simulink model "Pacemaker_Assignment_2_Final"  (R2018b)
settings: Solver=FixedStepAuto  StartTime=0.0  StopTime=inf  FixedStep=1e-3  RelTol=1e-3  EnableMultiTasking=on
undefined symbols (not defined in the file): D0, D1, D10, D11, D12, D13, D2, D3, D4, D5, D6, D7, D8, D9, PTA0, PTA1, PTA2, PTB23, PTB9, PTC16, PTC17, PTC2, PTC3, PTC4, PTD0, PTD1, PTD2, PTD3
libraries: frdmk64flib x20, dspstat3 x1
(part 1 of 2)
settings Model: EnablePacing=on  ExtModeTrigDuration=5  Creator=joelh  LastModifiedBy=joelh
settings OptimizationCC: EnhancedBackFolding=on  PassReuseOutputArgsAs=Individual arguments  MaxStackSize=64  OptimizeBlockOrder=speed  DifferentSizesBufferReuse=on  OptimizationCustomize=off
settings DebuggingCC: ParameterTunabilityLossMsg=error
settings HardwareCC: ProdBitPerPointer=32  ProdBitPerSizeT=32  ProdBitPerPtrDiffT=32  ProdLargestAtomicInteger=Long  ProdLargestAtomicFloat=Double  ProdWordSize=32  ProdHWDeviceType=ARM Compatible->ARM Cortex
settings SFSimCC: MATLABDynamicMemAlloc=off
settings RTWCC: SystemTargetFile=ert.tlc  HardwareBoard=NXP FRDM-K64F  TLCOptions="-aInlineSetEventsForThisBaseRateFcn=TLC_FALSE -aSuppressMultiTaskScheduler=TLC_FALSE  -aRateBasedStepFcn=0"  TemplateMakefile=ert_default_tmf  GenerateReport=on  Toolchain=GNU Tools for ARM Embedded Processors  IncludeHyperlinkInReport=on  LaunchReport=on  GenerateTraceInfo=on  GenerateTraceReport=on  GenerateTraceReportSl=on  GenerateTraceReportSf=on  GenerateTraceReportEml=on
settings CodeAppCC: ForceParamTrailComments=on  IgnoreCustomStorageClasses=off  OperatorAnnotations=on  SimulinkDataObjDesc=on  SFDataObjDesc=on  InsertBlockDesc=on

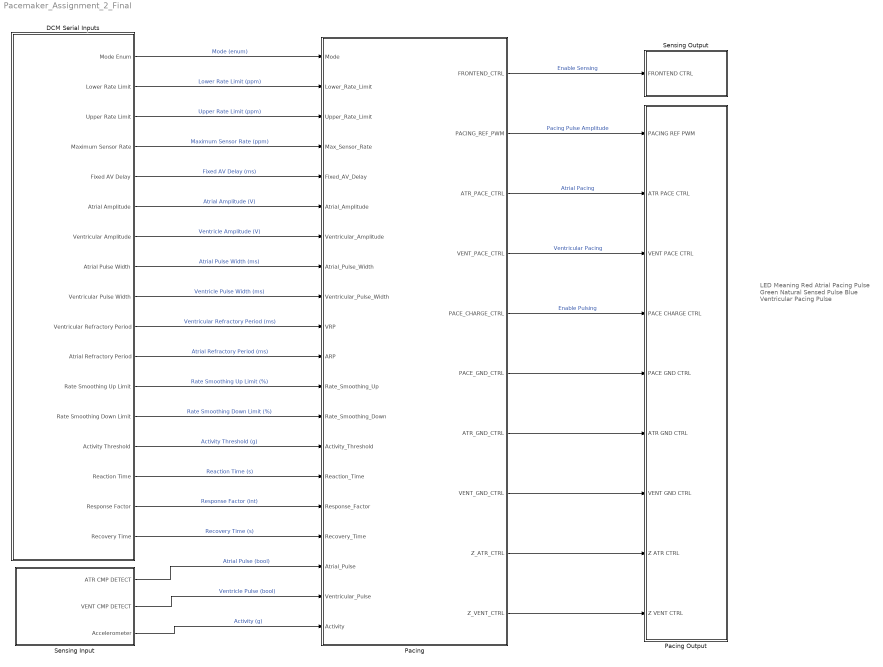
== system Pacemaker_Assignment_2_Final ==
  note: LED
      | Meaning
      |
      | Red
      | Atrial Pacing Pulse
      |
      | Green
      | Natural Sensed Pulse
      |
      | Blue
      | Ventricular Pacing Pulse
  DCM Serial Inputs : Subsystem
  Pacing : Stateflow chart  TreatAsAtomicUnit=on
  Pacing Output : Subsystem
  Sensing Input : Subsystem
  Sensing Output : Subsystem
  wires:
  DCM Serial Inputs/1(Mode Enum) -> Pacing/1(Mode)  "Mode (enum)"
  DCM Serial Inputs/2(Lower Rate Limit) -> Pacing/2(Lower_Rate_Limit)  "Lower Rate Limit (ppm)"
  DCM Serial Inputs/3(Upper Rate Limit) -> Pacing/3(Upper_Rate_Limit)  "Upper Rate Limit (ppm)"
  DCM Serial Inputs/4(Maximum Sensor Rate) -> Pacing/4(Max_Sensor_Rate)  "Maximum Sensor Rate (ppm)"
  DCM Serial Inputs/5(Fixed AV Delay) -> Pacing/5(Fixed_AV_Delay)  "Fixed AV Delay (ms)"
  DCM Serial Inputs/6(Atrial Amplitude) -> Pacing/6(Atrial_Amplitude)  "Atrial Amplitude (V)"
  DCM Serial Inputs/7(Ventricular Amplitude) -> Pacing/7(Ventricular_Amplitude)  "Ventricle Amplitude (V)"
  DCM Serial Inputs/8(Atrial Pulse Width) -> Pacing/8(Atrial_Pulse_Width)  "Atrial Pulse Width (ms)"
  DCM Serial Inputs/9(Ventricular Pulse Width) -> Pacing/9(Ventricular_Pulse_Width)  "Ventricle Pulse Width (ms)"
  DCM Serial Inputs/10(Ventricular Refractory Period) -> Pacing/10(VRP)  "Ventricular Refractory Period (ms)"
  DCM Serial Inputs/11(Atrial Refractory Period) -> Pacing/11(ARP)  "Atrial Refractory Period (ms)"
  DCM Serial Inputs/12(Rate Smoothing Up Limit) -> Pacing/12(Rate_Smoothing_Up)  "Rate Smoothing Up Limit (%)"
  DCM Serial Inputs/13(Rate Smoothing Down Limit) -> Pacing/13(Rate_Smoothing_Down)  "Rate Smoothing Down Limit (%)"
  DCM Serial Inputs/14(Activity Threshold) -> Pacing/14(Activity_Threshold)  "Activity Threshold (g)"
  DCM Serial Inputs/15(Reaction Time) -> Pacing/15(Reaction_Time)  "Reaction Time (s)"
  DCM Serial Inputs/16(Response Factor) -> Pacing/16(Response_Factor)  "Response Factor (int)"
  DCM Serial Inputs/17(Recovery Time) -> Pacing/17(Recovery_Time)  "Recovery Time (s)"
  Sensing Input/1(ATR CMP DETECT) -> Pacing/18(Atrial_Pulse)  "Atrial Pulse (bool)"
  Sensing Input/2(VENT CMP DETECT) -> Pacing/19(Ventricular_Pulse)  "Ventricle Pulse (bool)"
  Sensing Input/3(Accelerometer) -> Pacing/20(Activity)  "Activity (g)"
  Pacing/1(FRONTEND_CTRL) -> Sensing Output/1(FRONTEND CTRL)  "Enable Sensing"
  Pacing/2(PACING_REF_PWM) -> Pacing Output/1(PACING REF PWM)  "Pacing Pulse Amplitude"
  Pacing/3(ATR_PACE_CTRL) -> Pacing Output/2(ATR PACE CTRL)  "Atrial Pacing"
  Pacing/4(VENT_PACE_CTRL) -> Pacing Output/3(VENT PACE CTRL)  "Ventricular Pacing"
  Pacing/5(PACE_CHARGE_CTRL) -> Pacing Output/4(PACE CHARGE CTRL)  "Enable Pulsing"
  Pacing/6(PACE_GND_CTRL) -> Pacing Output/5(PACE GND CTRL)
  Pacing/7(ATR_GND_CTRL) -> Pacing Output/6(ATR GND CTRL)
  Pacing/8(VENT_GND_CTRL) -> Pacing Output/7(VENT GND CTRL)
  Pacing/9(Z_ATR_CTRL) -> Pacing Output/8(Z ATR CTRL)
  Pacing/10(Z_VENT_CTRL) -> Pacing Output/9(Z VENT CTRL)

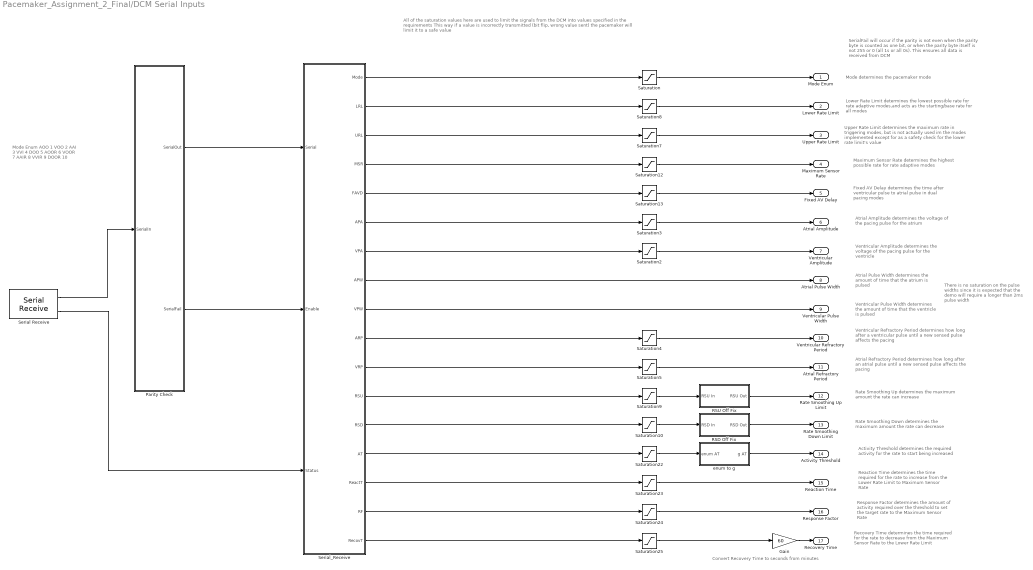
== system Pacemaker_Assignment_2_Final/DCM Serial Inputs ==
  note: Convert Recovery Time to seconds from minutes
  note: Recovery Time determines the time required for the rate to decrease from
      | the Maximum Sensor Rate to the Lower Rate Limit
  note: Response Factor determines the amount of activity required over the threshold to set the target rate to the Maximum Sensor Rate
  note: Reaction Time determines the time required for the rate to increase from the Lower Rate Limit to Maximum Sensor Rate
  note: Activity Threshold determines the required activity for the rate to start being increased
  note: Rate Smoothing Up determines the maximum amount the rate can increase
  note: Ventricular Refractory Period determines how long after a ventricular pulse until a new sensed pulse affects the pacing
  note: There is no saturation on the pulse widths since it is expected that
      | the demo will require a longer than 2ms pulse width
  note: Atrial Pulse Width determines the amount of time that the atrium is pulsed
  note: Atrial Amplitude determines the voltage of the pacing pulse for the atrium
  note: Fixed AV Delay determines the time after ventricular pulse to atrial pulse in
      | dual pacing modes
  note: Maximum Sensor Rate determines the highest possible rate for rate adaptive modes
  note: Upper Rate Limit determines the maximum rate in triggering modes, but is not actually used im the modes implemented except for as a safety check for the lower rate limit's value
  note: Lower Rate Limit determines the lowest possible rate for rate adaptive modes,and acts as the starting/base rate for all modes
  note: SerialFail will occur if the parity is not even when the parity byte is counted as one bit, or when the parity byte itself is not 255 or 0 (all 1s or all 0s). This ensures all data is received from DCM
  note: Mode determines the pacemaker mode
  note: All of the saturation values here are used to limit the signals from the DCM into values specified in the requirements
      | This way if a value is incorrectly transmitted (bit flip, wrong value sent) the pacemaker will limit it to a safe value
  note: Mode
      | Enum
      |
      | AOO
      | 1
      |
      | VOO
      | 2
      |
      | AAI
      | 3
      |
      | VVI
      | 4
      |
      | DOO
      | 5
      |
      | AOOR
      | 6
      |
      | VOOR
      | 7
      |
      | AAIR
      | 8
      |
      | VVIR
      | 9
      |
      | DOOR
      | 10
  note: Ventricular Amplitude determines the voltage of the pacing pulse for the ventricle
  note: Ventricular Pulse Width determines the amount of time that the ventricle is pulsed
  note: Atrial Refractory Period determines how long after an atrial pulse until a new sensed pulse affects the pacing
  note: Rate Smoothing Down determines the maximum amount the rate can decrease
  Gain : Gain  Gain=60
  Parity Check : MATLAB Function  TreatAsAtomicUnit=on
  RSD Off Fix : Subsystem
  RSU Off Fix : Subsystem
  Saturation : Saturate  UpperLimit=10  LowerLimit=0
  Saturation10 : Saturate  UpperLimit=25  LowerLimit=0
  Saturation12 : Saturate  UpperLimit=175  LowerLimit=50
  Saturation13 : Saturate  UpperLimit=300  LowerLimit=70
  Saturation2 : Saturate  UpperLimit=5  LowerLimit=0
  Saturation22 : Saturate  UpperLimit=7  LowerLimit=1
  Saturation23 : Saturate  UpperLimit=50  LowerLimit=10
  Saturation24 : Saturate  UpperLimit=16  LowerLimit=1
  Saturation25 : Saturate  UpperLimit=16  LowerLimit=2
  Saturation3 : Saturate  UpperLimit=5  LowerLimit=0
  Saturation4 : Saturate  UpperLimit=500  LowerLimit=150
  Saturation5 : Saturate  UpperLimit=500  LowerLimit=150
  Saturation7 : Saturate  UpperLimit=175  LowerLimit=50
  Saturation8 : Saturate  UpperLimit=175  LowerLimit=30
  Saturation9 : Saturate  UpperLimit=25  LowerLimit=0
  Serial Receive : frdmk64flib/Serial Receive  SCIModule=0  Baudrate=uint32(9600)  Parity=None  StopBits=1  HardwareFlowControl=None  ByteOrder=LittleEndian  DataType=uint8  DataLength=18  BlockingMode=off  OutputStatus=on  SampleTime=-1
      settings: SourceProductName=Simulink Coder Support Package for NXP FRDM-K64F Board
  Serial_Receive : Stateflow chart  TreatAsAtomicUnit=on
  enum to g : Subsystem
  Mode Enum : Outport
  Lower Rate Limit : Outport  Port=2
  Upper Rate Limit : Outport  Port=3
  Maximum Sensor Rate : Outport  Port=4
  Fixed AV Delay : Outport  Port=5
  Atrial Amplitude : Outport  Port=6
  Ventricular Amplitude : Outport  Port=7
  Atrial Pulse Width : Outport  Port=8
  Ventricular Pulse Width : Outport  Port=9
  Ventricular Refractory Period : Outport  Port=10
  Atrial Refractory Period : Outport  Port=11
  Rate Smoothing Up Limit : Outport  Port=12
  Rate Smoothing Down Limit : Outport  Port=13
  Activity Threshold : Outport  Port=14
  Reaction Time : Outport  Port=15
  Response Factor : Outport  Port=16
  Recovery Time : Outport  Port=17
  wires:
  Serial_Receive/6(APA) -> Saturation3/1
  Serial_Receive/2(LRL) -> Saturation8/1
  Serial_Receive/7(VPA) -> Saturation2/1
  Serial_Receive/3(URL) -> Saturation7/1
  Serial_Receive/10(ARP) -> Saturation4/1
  Serial_Receive/11(VRP) -> Saturation5/1
  Serial_Receive/12(RSU) -> Saturation9/1
  Serial_Receive/13(RSD) -> Saturation10/1
  Saturation2/1 -> Ventricular Amplitude/1
  Saturation3/1 -> Atrial Amplitude/1
  Saturation4/1 -> Ventricular Refractory Period/1
  Saturation5/1 -> Atrial Refractory Period/1
  Saturation7/1 -> Upper Rate Limit/1
  Saturation8/1 -> Lower Rate Limit/1
  Saturation9/1 -> RSU Off Fix/1(RSU In)
  Saturation10/1 -> RSD Off Fix/1(RSD In)
  Serial_Receive/5(FAVD) -> Saturation13/1
  Serial_Receive/4(MSR) -> Saturation12/1
  Serial_Receive/14(AT) -> Saturation22/1
  Serial_Receive/15(ReactT) -> Saturation23/1
  Serial_Receive/16(RF) -> Saturation24/1
  Serial_Receive/17(RecovT) -> Saturation25/1
  Saturation22/1 -> enum to g/1(enum AT)
  Serial_Receive/1(Mode) -> Saturation/1
  Gain/1 -> Recovery Time/1
  Saturation12/1 -> Maximum Sensor Rate/1
  Saturation13/1 -> Fixed AV Delay/1
  Serial_Receive/8(APW) -> Atrial Pulse Width/1
  Serial_Receive/9(VPW) -> Ventricular Pulse Width/1
  Saturation23/1 -> Reaction Time/1
  Saturation24/1 -> Response Factor/1
  Saturation25/1 -> Gain/1
  enum to g/1(g AT) -> Activity Threshold/1
  Saturation/1 -> Mode Enum/1
  Parity Check/1(SerialOut) -> Serial_Receive/1(Serial)
  Serial Receive/1 -> Parity Check/1(SerialIn)
  Serial Receive/2 -> Serial_Receive/3(Status)
  Parity Check/2(SerialFail) -> Serial_Receive/2(Enable)
  RSU Off Fix/1(RSU Out) -> Rate Smoothing Up Limit/1
  RSD Off Fix/1(RSD Out) -> Rate Smoothing Down Limit/1

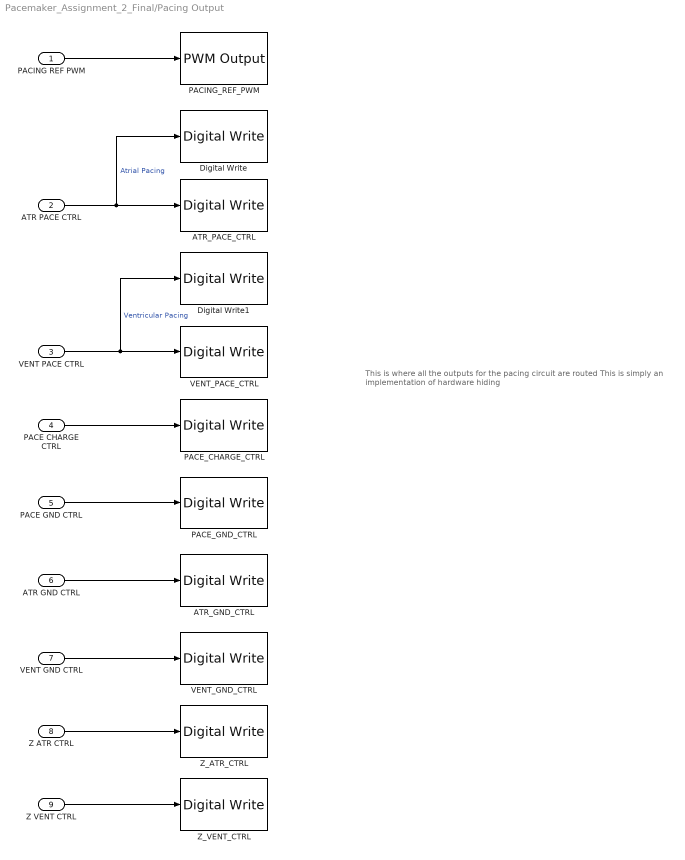
== system Pacemaker_Assignment_2_Final/Pacing Output ==
  note: This is where all the outputs for the pacing circuit are routed
      | This is simply an implementation of hardware hiding
  PACING REF PWM : Inport
  ATR PACE CTRL : Inport  Port=2
  VENT PACE CTRL : Inport  Port=3
  PACE CHARGE CTRL : Inport  Port=4
  PACE GND CTRL : Inport  Port=5
  ATR GND CTRL : Inport  Port=6
  VENT GND CTRL : Inport  Port=7
  Z ATR CTRL : Inport  Port=8
  Z VENT CTRL : Inport  Port=9
  ATR_GND_CTRL : frdmk64flib/Digital Write  Whichpin=PTD2 (D11)
      settings: SourceProductName=Simulink Coder Support Package for NXP FRDM-K64F Board
  ATR_PACE_CTRL : frdmk64flib/Digital Write  Whichpin=PTA0 (D8)
      settings: SourceProductName=Simulink Coder Support Package for NXP FRDM-K64F Board
  Digital Write : frdmk64flib/Digital Write  Whichpin=RED_LED
      settings: SourceProductName=Simulink Coder Support Package for NXP FRDM-K64F Board
  Digital Write1 : frdmk64flib/Digital Write  Whichpin=BLUE_LED
      settings: SourceProductName=Simulink Coder Support Package for NXP FRDM-K64F Board
  PACE_CHARGE_CTRL : frdmk64flib/Digital Write  Whichpin=PTB9 (D2)
      settings: SourceProductName=Simulink Coder Support Package for NXP FRDM-K64F Board
  PACE_GND_CTRL : frdmk64flib/Digital Write  Whichpin=PTD0 (D10)
      settings: SourceProductName=Simulink Coder Support Package for NXP FRDM-K64F Board
  PACING_REF_PWM : frdmk64flib/PWM Output  Whichpin=PTA2 (D5)  InitialFrequency=2000  InitialDutyCycle=0
      settings: SourceProductName=Simulink Coder Support Package for NXP FRDM-K64F Board
  VENT_GND_CTRL : frdmk64flib/Digital Write  Whichpin=PTD3 (D12)
      settings: SourceProductName=Simulink Coder Support Package for NXP FRDM-K64F Board
  VENT_PACE_CTRL : frdmk64flib/Digital Write  Whichpin=PTC4 (D9)
      settings: SourceProductName=Simulink Coder Support Package for NXP FRDM-K64F Board
  Z_ATR_CTRL : frdmk64flib/Digital Write  Whichpin=PTB23 (D4)
      settings: SourceProductName=Simulink Coder Support Package for NXP FRDM-K64F Board
  Z_VENT_CTRL : frdmk64flib/Digital Write  Whichpin=PTC3 (D7)
      settings: SourceProductName=Simulink Coder Support Package for NXP FRDM-K64F Board
  wires:
  ATR GND CTRL/1 -> ATR_GND_CTRL/1
  VENT GND CTRL/1 -> VENT_GND_CTRL/1
  ATR PACE CTRL/1 -> Digital Write/1, ATR_PACE_CTRL/1  "Atrial Pacing"
  PACE GND CTRL/1 -> PACE_GND_CTRL/1
  PACING REF PWM/1 -> PACING_REF_PWM/1
  PACE CHARGE CTRL/1 -> PACE_CHARGE_CTRL/1
  Z ATR CTRL/1 -> Z_ATR_CTRL/1
  Z VENT CTRL/1 -> Z_VENT_CTRL/1
  VENT PACE CTRL/1 -> Digital Write1/1, VENT_PACE_CTRL/1  "Ventricular Pacing"

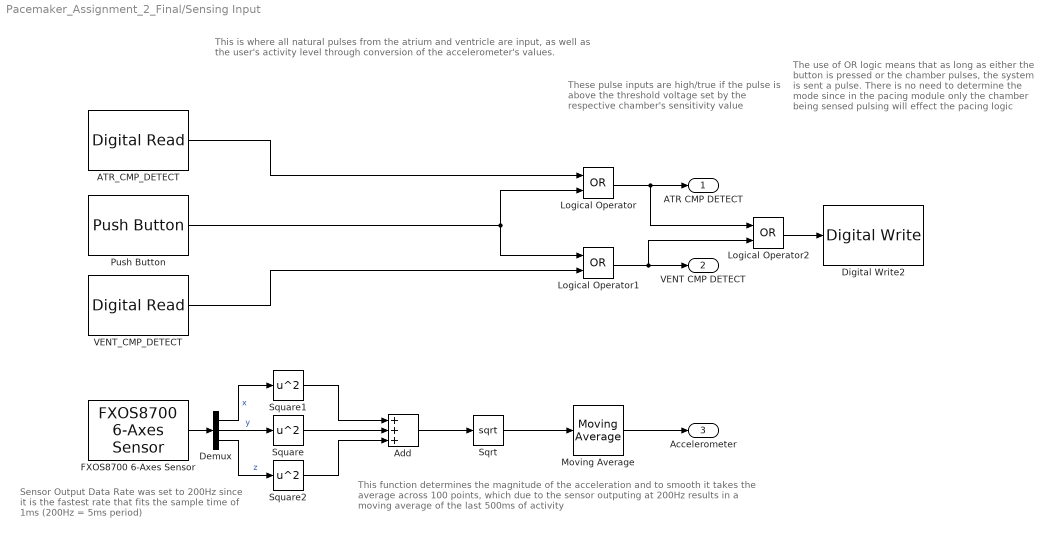
== system Pacemaker_Assignment_2_Final/Sensing Input ==
  note: Sensor Output Data Rate was set to 200Hz since it is the fastest rate that fits the sample time of 1ms (200Hz = 5ms period)
  note: This function determines the magnitude of the acceleration and to smooth it takes the average across 100 points, which due to the sensor outputing at 200Hz results in a moving average of the last 500ms of activity
  note: This is where all natural pulses from the atrium and ventricle are input, as well
      | as the user's activity level through conversion of the accelerometer's values.
  note: The use of OR logic means that as long as either the button is pressed or the chamber pulses, the system is sent a pulse. There is no need to determine the mode since in the pacing module only the chamber being sensed pulsing will effect the pacing logic
  note: These pulse inputs are high/true if the pulse is above the threshold voltage set by the respective chamber's sensitivity value
  ATR_CMP_DETECT : frdmk64flib/Digital Read  Whichpin=PTC16 (D0)  SampleTime=-1
      settings: SourceProductName=Simulink Coder Support Package for NXP FRDM-K64F Board
  Add : Sum  Inputs=3
  Demux : Demux  Outputs=3
  Digital Write2 : frdmk64flib/Digital Write  Whichpin=GREEN_LED
      settings: SourceProductName=Simulink Coder Support Package for NXP FRDM-K64F Board
  FXOS8700 6-Axes Sensor : frdmk64flib/FXOS8700 6-Axes Sensor  Activesensor=Accelerometer only  ODR=200Hz  HybridODR=400Hz  Accelfullrange=-4g to +4g  SampleTime=-1
      settings: SourceProductName=Simulink Coder Support Package for NXP FRDM-K64F Board
  Logical Operator : Logic  Operator=OR  AllPortsSameDT=off  OutDataTypeStr=boolean
  Logical Operator1 : Logic  Operator=OR  AllPortsSameDT=off  OutDataTypeStr=boolean
  Logical Operator2 : Logic  Operator=OR  AllPortsSameDT=off  OutDataTypeStr=boolean
  Moving Average : dspstat3/Moving Average  Method=Sliding window  ForgettingFactorPort=off  SpecifyWindowLength=on  WindowLength=100  ForgettingFactor=0.9  SimulateUsing=Code generation
  "Push Button " : frdmk64flib/Push Button  Whichswitch=SW3  SampleTime1=-1
      settings: SourceProductName=Simulink Coder Support Package for NXP FRDM-K64F Board
  Sqrt : Sqrt  SaturateOnIntegerOverflow=on
  Square : Math  Operator=square  SaturateOnIntegerOverflow=on
  Square1 : Math  Operator=square  SaturateOnIntegerOverflow=on
  Square2 : Math  Operator=square  SaturateOnIntegerOverflow=on
  VENT_CMP_DETECT : frdmk64flib/Digital Read  Whichpin=PTC17 (D1)  SampleTime=-1
      settings: SourceProductName=Simulink Coder Support Package for NXP FRDM-K64F Board
  ATR CMP DETECT : Outport
  VENT CMP DETECT : Outport  Port=2
  Accelerometer : Outport  Port=3
  wires:
  Logical Operator1/1 -> Logical Operator2/2, VENT CMP DETECT/1
  Logical Operator/1 -> Logical Operator2/1, ATR CMP DETECT/1
  ATR_CMP_DETECT/1 -> Logical Operator/1
  "Push Button "/1 -> Logical Operator1/1, Logical Operator/2
  VENT_CMP_DETECT/1 -> Logical Operator1/2
  Moving Average/1 -> Accelerometer/1
  Demux/2 -> Square/1  "y"
  Demux/1 -> Square1/1  "x"
  Add/1 -> Sqrt/1
  FXOS8700 6-Axes Sensor/1 -> Demux/1
  Square/1 -> Add/2
  Square1/1 -> Add/1
  Square2/1 -> Add/3
  Demux/3 -> Square2/1  "z"
  Sqrt/1 -> Moving Average/1
  Logical Operator2/1 -> Digital Write2/1

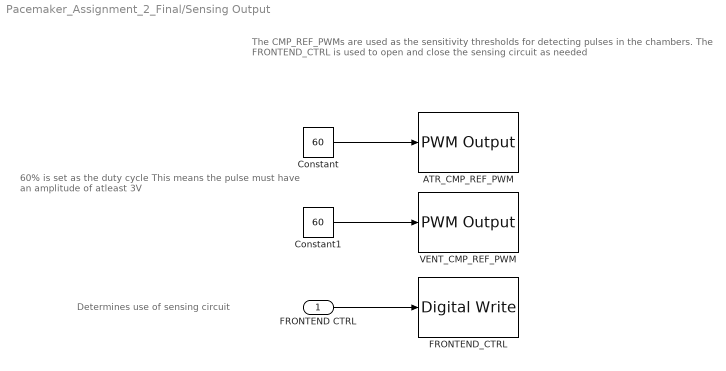
== system Pacemaker_Assignment_2_Final/Sensing Output ==
  note: 60% is set as the duty cycle
      | This means the pulse must have an amplitude of atleast 3V
  note: The CMP_REF_PWMs are used as the sensitivity thresholds for detecting pulses in the chambers.
      | The FRONTEND_CTRL is used to open and close the sensing circuit as needed
  note: Determines use of sensing circuit
  FRONTEND CTRL : Inport
  ATR_CMP_REF_PWM : frdmk64flib/PWM Output  Whichpin=PTC2 (D6)  InitialFrequency=2000  InitialDutyCycle=0
      settings: SourceProductName=Simulink Coder Support Package for NXP FRDM-K64F Board
  Constant : Constant  Value=60
  Constant1 : Constant  Value=60
  FRONTEND_CTRL : frdmk64flib/Digital Write  Whichpin=PTD1 (D13)
      settings: SourceProductName=Simulink Coder Support Package for NXP FRDM-K64F Board
  VENT_CMP_REF_PWM : frdmk64flib/PWM Output  Whichpin=PTA1 (D3)  InitialFrequency=2000  InitialDutyCycle=0
      settings: SourceProductName=Simulink Coder Support Package for NXP FRDM-K64F Board
  wires:
  FRONTEND CTRL/1 -> FRONTEND_CTRL/1
  Constant/1 -> ATR_CMP_REF_PWM/1
  Constant1/1 -> VENT_CMP_REF_PWM/1

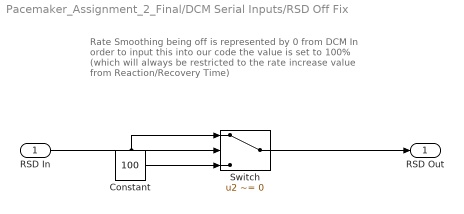
== system Pacemaker_Assignment_2_Final/DCM Serial Inputs/RSD Off Fix ==
  note: Rate Smoothing being off is represented by 0 from DCM
      | In order to input this into our code the value is set to 100% (which will always be restricted to the
      | rate increase value from Reaction/Recovery Time)
  RSD In : Inport
  Constant : Constant  Value=100
  Switch : Switch  Criteria=u2 ~= 0
  RSD Out : Outport
  wires:
  Constant/1 -> Switch/3
  RSD In/1 -> Switch/1, Switch/2
  Switch/1 -> RSD Out/1

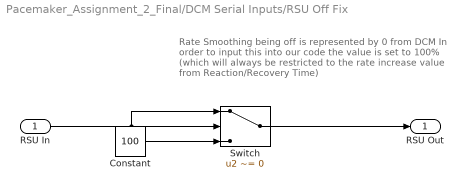
== system Pacemaker_Assignment_2_Final/DCM Serial Inputs/RSU Off Fix ==
  note: Rate Smoothing being off is represented by 0 from DCM
      | In order to input this into our code the value is set to 100% (which will always be restricted to the
      | rate increase value from Reaction/Recovery Time)
  RSU In : Inport
  Constant : Constant  Value=100
  Switch : Switch  Criteria=u2 ~= 0
  RSU Out : Outport
  wires:
  RSU In/1 -> Switch/1, Switch/2
  Switch/1 -> RSU Out/1
  Constant/1 -> Switch/3

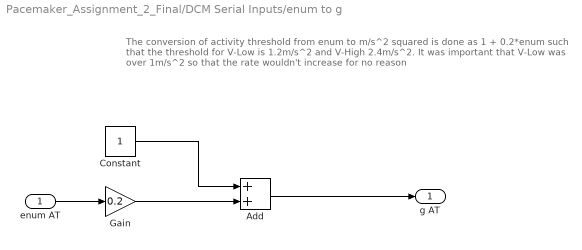
== system Pacemaker_Assignment_2_Final/DCM Serial Inputs/enum to g ==
  note: The conversion of activity threshold from enum to m/s^2 squared is done as
      | 1 + 0.2*enum such that the threshold for V-Low is 1.2m/s^2 and V-High 2.4m/s^2.
      | It was important that V-Low was over 1m/s^2 so that the rate wouldn't increase for no reason
  enum AT : Inport
  Add : Sum
  Constant : Constant
  Gain : Gain  Gain=0.2
  g AT : Outport
  wires:
  enum AT/1 -> Gain/1
  Gain/1 -> Add/2
  Add/1 -> g AT/1
  Constant/1 -> Add/1

== matlab function Pacemaker_Assignment_2_Final/DCM Serial Inputs/Parity Check ==
  data: SerialOut output uint8; SerialFail output boolean; SerialIn input
function [SerialOut, SerialFail]= Unpack(SerialIn)
%This is the serial checking and unpacking of the parameters from DCM
%Byte 1: Parity (SerialFail) Using Even parity
if (SerialIn(1) == 255) %Odd number of 1s in bytes 2-18
    numOnes = uint8(0);
    for i = 2:18 %every byte
        temp = SerialIn(i);
        for j = 1:8 %every bit
            numOnes = numOnes + uint8(bitget(temp,j));
        end
    end
    if (mod(numOnes,2)) %odd number of 1s
        SerialFail = false;
    else %even number of 1s
        SerialFail = true;
    end
        
elseif (SerialIn(1) == 0) %Even number of 1s in bytes 2-18
    numOnes = uint8(0);
    for i = 2:18 %every byte
        temp = SerialIn(i);
        for j = 1:8 %every bit
            numOnes = numOnes + uint8(bitget(temp,j));
        end
    end
    if (~mod(numOnes,2)) %even number of 1s
        SerialFail = false;
    else %odd number of 1s
        SerialFail = true;
    end
    
else %invalid parity
    SerialFail = true;
end
SerialOut = SerialIn;
end
